simulink model "power_balance"  (R2022a)
settings: Solver=VariableStepAuto  StartTime=0.0  StopTime=11  RelTol=1e-3
undefined symbols (not defined in the file): CA, f, g, i, i0, kt, m2, r
libraries: simulink x1
settings Model: DataDictionary=Vehicle_paramiter.sldd  Creator=cht  LastModifiedBy=cht

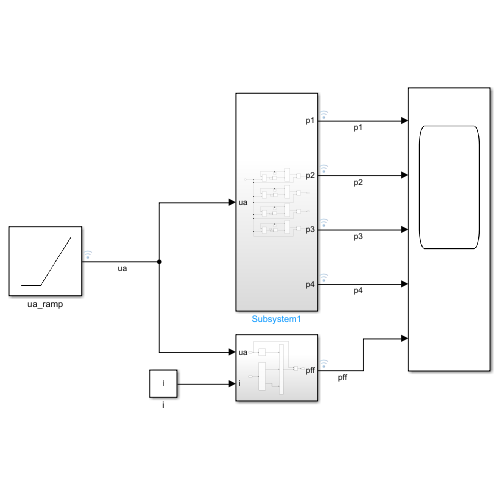
[thumbnail: Simulink's stored preview of the top-level diagram]
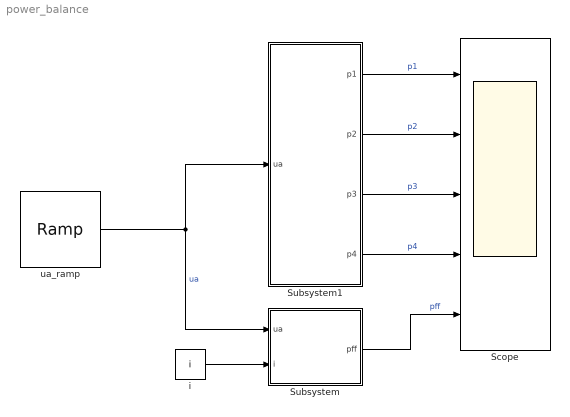
== system power_balance ==
  Scope : Scope  NumInputPorts=5
  Subsystem : Subsystem
  Subsystem1 : Subsystem
  i : Constant  Value=i
  ua_ramp : simulink/Sources/Ramp  slope=11  start=0  InitialOutput=0
  wires:
  ua_ramp/1 -> Subsystem1/1(ua), Subsystem/1(ua)  "ua"
  i/1 -> Subsystem/2(i)
  Subsystem1/1(p1) -> Scope/1  "p1"
  Subsystem/1(pff) -> Scope/5  "pff"
  Subsystem1/2(p2) -> Scope/2  "p2"
  Subsystem1/3(p3) -> Scope/3  "p3"
  Subsystem1/4(p4) -> Scope/4  "p4"

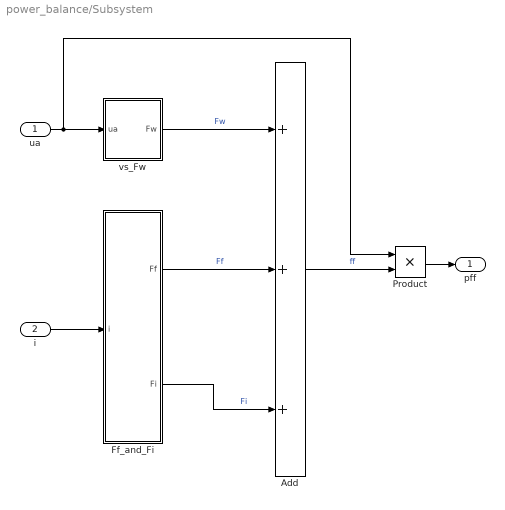
== system power_balance/Subsystem ==
  ua : Inport
  i : Inport  Port=2
  Add : Sum  Inputs=+++
  Ff_and_Fi : Subsystem
  Product : Product
  vs_Fw : Subsystem
  pff : Outport
  wires:
  Add/1 -> Product/2  "ff"
  vs_Fw/1(Fw) -> Add/1  "Fw"
  i/1 -> Ff_and_Fi/1(i)
  ua/1 -> Product/1, vs_Fw/1(ua)
  Ff_and_Fi/2(Fi) -> Add/3  "Fi"
  Ff_and_Fi/1(Ff) -> Add/2  "Ff"
  Product/1 -> pff/1

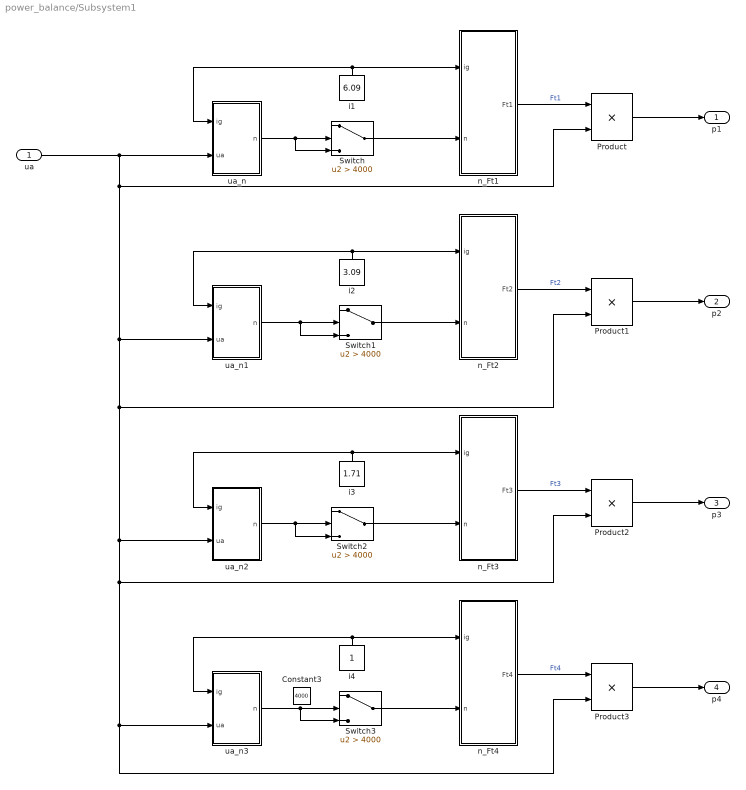
== system power_balance/Subsystem1 ==
  ua : Inport
  Constant3 : Constant  Value=4000
  Product{,1..3} (4 alike) : Product
  Switch{,1..3} (4 alike) : Switch  Criteria=u2 > Threshold  Threshold=4000  SaturateOnIntegerOverflow=off  InputSameDT=off
  i1 : Constant  Value=6.09
  i2 : Constant  Value=3.09
  i3 : Constant  Value=1.71
  i4 : Constant
  n_Ft1 : Subsystem
  n_Ft2 : Subsystem
  n_Ft3 : Subsystem
  n_Ft4 : Subsystem
  ua_n : Subsystem
  ua_n1 : Subsystem
  ua_n2 : Subsystem
  ua_n3 : Subsystem
  p1 : Outport
  p2 : Outport  Port=2
  p3 : Outport  Port=3
  p4 : Outport  Port=4
  wires:
  n_Ft4/1(Ft4) -> Product3/1  "Ft4"
  n_Ft2/1(Ft2) -> Product1/1  "Ft2"
  i1/1 -> ua_n/1(ig), n_Ft1/1(ig)
  ua/1 -> Product/2, Product1/2, Product2/2, Product3/2, ua_n3/2(ua), ua_n2/2(ua), ua_n1/2(ua), ua_n/2(ua)
  ua_n/1(n) -> Switch/2, Switch/3
  i2/1 -> n_Ft2/1(ig), ua_n1/1(ig)
  n_Ft1/1(Ft1) -> Product/1  "Ft1"
  n_Ft3/1(Ft3) -> Product2/1  "Ft3"
  i4/1 -> ua_n3/1(ig), n_Ft4/1(ig)
  i3/1 -> n_Ft3/1(ig), ua_n2/1(ig)
  Product/1 -> p1/1
  Product1/1 -> p2/1
  Product2/1 -> p3/1
  Product3/1 -> p4/1
  Switch/1 -> n_Ft1/2(n)
  ua_n2/1(n) -> Switch2/2, Switch2/3
  ua_n3/1(n) -> Switch3/2, Switch3/3
  Switch3/1 -> n_Ft4/2(n)
  Switch2/1 -> n_Ft3/2(n)
  ua_n1/1(n) -> Switch1/3, Switch1/2
  Switch1/1 -> n_Ft2/2(n)

== system power_balance/Subsystem/Ff_and_Fi ==
  i : Inport
  Subsystem : Subsystem
  Trigonometric Function : Trigonometry  Operator=atan
  Ff : Outport
  Fi : Outport  Port=2
  wires:
  i/1 -> Trigonometric Function/1
  Subsystem/1(Ff) -> Ff/1
  Trigonometric Function/1 -> Subsystem/1(angle)
  Subsystem/2(Fi) -> Fi/1

== system power_balance/Subsystem/vs_Fw ==
  ua : Inport
  Constant1 : Constant  Value=2
  Gain : Gain  Gain=CA/21.15
  Power : Math  Operator=pow
  Fw : Outport
  wires:
  Constant1/1 -> Power/2
  Gain/1 -> Fw/1
  ua/1 -> Power/1
  Power/1 -> Gain/1

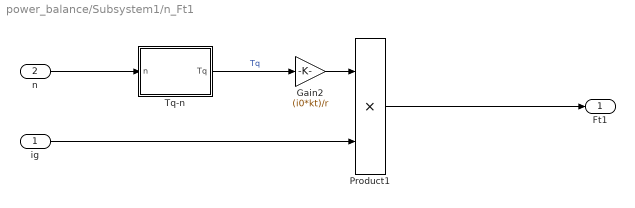
== system power_balance/Subsystem1/n_Ft1 ==
  ig : Inport
  n : Inport  Port=2
  Gain2 : Gain  Gain=(i0*kt)/r
  Product1 : Product
  Tq-n : MATLAB Function  TreatAsAtomicUnit=on
  Ft1 : Outport
  wires:
  Product1/1 -> Ft1/1
  ig/1 -> Product1/2
  Tq-n/1(Tq) -> Gain2/1  "Tq"
  n/1 -> Tq-n/1(n)
  Gain2/1 -> Product1/1

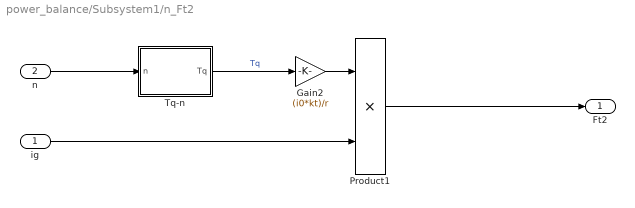
== system power_balance/Subsystem1/n_Ft2 ==
  ig : Inport
  n : Inport  Port=2
  Gain2 : Gain  Gain=(i0*kt)/r
  Product1 : Product
  Tq-n : MATLAB Function  TreatAsAtomicUnit=on
  Ft2 : Outport
  wires:
  Gain2/1 -> Product1/1
  n/1 -> Tq-n/1(n)
  Tq-n/1(Tq) -> Gain2/1  "Tq"
  ig/1 -> Product1/2
  Product1/1 -> Ft2/1

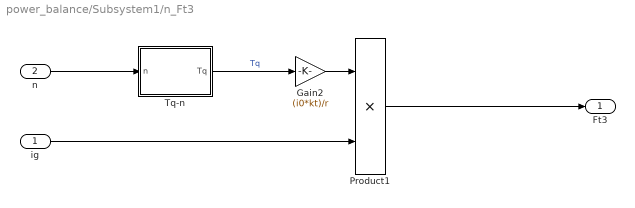
== system power_balance/Subsystem1/n_Ft3 ==
  ig : Inport
  n : Inport  Port=2
  Gain2 : Gain  Gain=(i0*kt)/r
  Product1 : Product
  Tq-n : MATLAB Function  TreatAsAtomicUnit=on
  Ft3 : Outport
  wires:
  Gain2/1 -> Product1/1
  n/1 -> Tq-n/1(n)
  Tq-n/1(Tq) -> Gain2/1  "Tq"
  ig/1 -> Product1/2
  Product1/1 -> Ft3/1

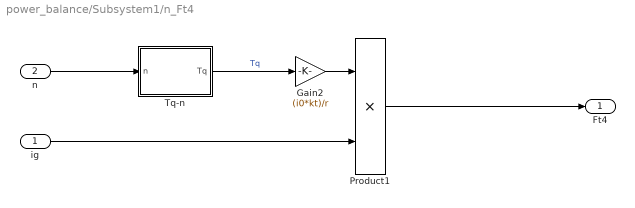
== system power_balance/Subsystem1/n_Ft4 ==
  ig : Inport
  n : Inport  Port=2
  Gain2 : Gain  Gain=(i0*kt)/r
  Product1 : Product
  Tq-n : MATLAB Function  TreatAsAtomicUnit=on
  Ft4 : Outport
  wires:
  Product1/1 -> Ft4/1
  ig/1 -> Product1/2
  Tq-n/1(Tq) -> Gain2/1  "Tq"
  n/1 -> Tq-n/1(n)
  Gain2/1 -> Product1/1

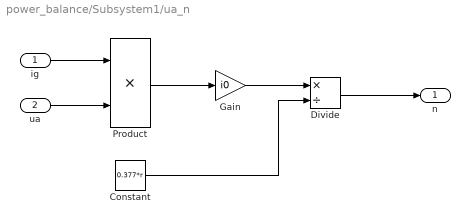
== system power_balance/Subsystem1/ua_n ==
  ig : Inport
  ua : Inport  Port=2
  Constant : Constant  Value=0.377*r
  Divide : Product  Inputs=*/
  Gain : Gain  Gain=i0
  Product : Product
  n : Outport
  wires:
  ua/1 -> Product/2
  Product/1 -> Gain/1
  Divide/1 -> n/1
  Constant/1 -> Divide/2
  Gain/1 -> Divide/1
  ig/1 -> Product/1

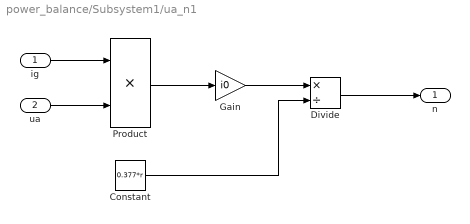
== system power_balance/Subsystem1/ua_n1 ==
  ig : Inport
  ua : Inport  Port=2
  Constant : Constant  Value=0.377*r
  Divide : Product  Inputs=*/
  Gain : Gain  Gain=i0
  Product : Product
  n : Outport
  wires:
  ig/1 -> Product/1
  Gain/1 -> Divide/1
  Constant/1 -> Divide/2
  Divide/1 -> n/1
  Product/1 -> Gain/1
  ua/1 -> Product/2

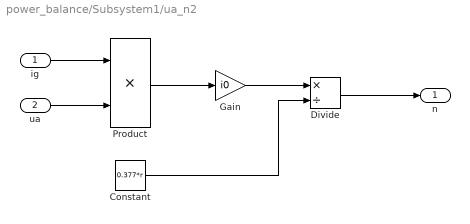
== system power_balance/Subsystem1/ua_n2 ==
  ig : Inport
  ua : Inport  Port=2
  Constant : Constant  Value=0.377*r
  Divide : Product  Inputs=*/
  Gain : Gain  Gain=i0
  Product : Product
  n : Outport
  wires:
  ig/1 -> Product/1
  Gain/1 -> Divide/1
  Constant/1 -> Divide/2
  Divide/1 -> n/1
  Product/1 -> Gain/1
  ua/1 -> Product/2

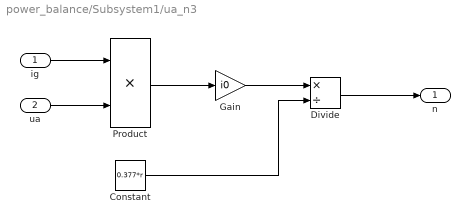
== system power_balance/Subsystem1/ua_n3 ==
  ig : Inport
  ua : Inport  Port=2
  Constant : Constant  Value=0.377*r
  Divide : Product  Inputs=*/
  Gain : Gain  Gain=i0
  Product : Product
  n : Outport
  wires:
  ua/1 -> Product/2
  Product/1 -> Gain/1
  Divide/1 -> n/1
  Constant/1 -> Divide/2
  Gain/1 -> Divide/1
  ig/1 -> Product/1

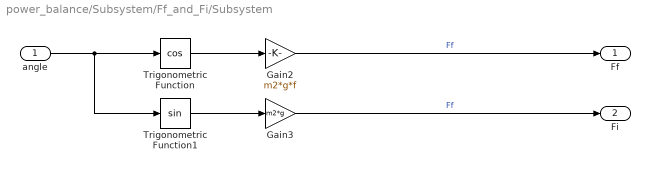
== system power_balance/Subsystem/Ff_and_Fi/Subsystem ==
  angle : Inport
  Gain2 : Gain  Gain=m2*g*f
  Gain3 : Gain  Gain=m2*g
  Trigonometric Function : Trigonometry  Operator=cos
  Trigonometric Function1 : Trigonometry
  Ff : Outport
  Fi : Outport  Port=2
  wires:
  Gain3/1 -> Fi/1  "Ff"
  angle/1 -> Trigonometric Function1/1, Trigonometric Function/1
  Trigonometric Function1/1 -> Gain3/1
  Trigonometric Function/1 -> Gain2/1
  Gain2/1 -> Ff/1  "Ff"

== matlab function power_balance/Subsystem1/n_Ft2/Tq-n ==
  data: n input; Tq output
function Tq = fcn(n)
%#codegen

Tq = -19.313+295.27*(n/1000)-165.44*(n/1000)^2+40.874*(n/1000)^3-3.8445*(n/1000)^4;

== matlab function power_balance/Subsystem1/n_Ft3/Tq-n ==
  data: n input; Tq output
function Tq = fcn(n)
%#codegen

Tq = -19.313+295.27*(n/1000)-165.44*(n/1000)^2+40.874*(n/1000)^3-3.8445*(n/1000)^4;

== matlab function power_balance/Subsystem1/n_Ft4/Tq-n ==
  data: n input; Tq output
function Tq = fcn(n)
%#codegen

Tq = -19.313+295.27*(n/1000)-165.44*(n/1000)^2+40.874*(n/1000)^3-3.8445*(n/1000)^4;

== matlab function power_balance/Subsystem1/n_Ft1/Tq-n ==
  data: n input; Tq output
function Tq = fcn(n)
%#codegen

Tq = -19.313+295.27*(n/1000)-165.44*(n/1000)^2+40.874*(n/1000)^3-3.8445*(n/1000)^4;
